simulink model "frontal"  (R2022b)
settings: Solver=VariableStepAuto  StartTime=0.0  StopTime=2  RelTol=1e-3
undefined symbols (not defined in the file or in its folder): Kx, x0, xr
settings Model: Creator=mmaximo  LastModifiedBy=danie
settings SolverCC: AlgebraicLoopSolver=TrustRegion
settings DebuggingCC: UnconnectedInputMsg=warning  UnconnectedOutputMsg=warning  UnconnectedLineMsg=warning  SFMachineParentedDataDiag=warning
settings ModelReferenceCC: EnableRefExpFcnMdlSchedulingChecks=on
settings RTWCC: DLArmComputeVersion=19.05

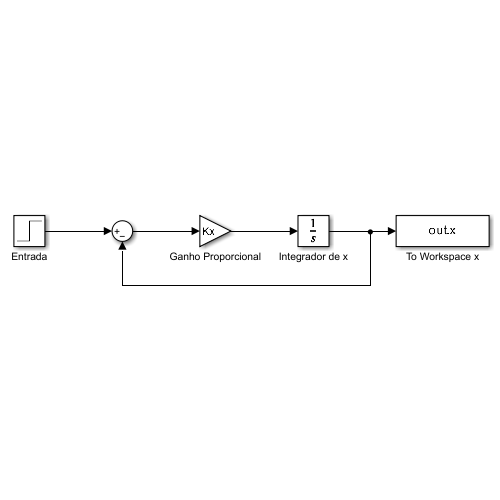
[thumbnail: Simulink's stored preview of the top-level diagram]
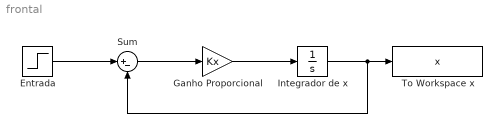
== system frontal ==
  Entrada : Step  Time=0  Before=x0  After=xr  SampleTime=0
  Ganho Proporcional : Gain  Gain=Kx
  Integrador de x : Integrator
  Sum : Sum  Inputs=|+-
  To Workspace x : ToWorkspace  VariableName=x  SaveFormat=Structure With Time  SampleTime=-1
  wires:
  Integrador de x/1 -> Sum/2, To Workspace x/1
  Ganho Proporcional/1 -> Integrador de x/1
  Sum/1 -> Ganho Proporcional/1
  Entrada/1 -> Sum/1
